simulink model "LAB_Stima_e_Controllo_Lez_5_Pendolo_Inverso_Simulink"  (R2018a)
settings: Solver=VariableStepAuto  StartTime=0.0  StopTime=10.0  RelTol=1e-3
values from neighbouring files (symbols this model uses):
  g = 9.81    [LAB_Stima_e_Controllo_Lez_2_Sistema_Idraulico.m]    (also in LAB_Stima_e_Controllo_Lez_4_Pendolo_Inverso.m)
  K2 = place(A,B,p2)    [LAB_Stima_e_Controllo_Lez_1_Motore_Corrente_Continua.m]    (also in LAB_Stima_e_Controllo_Lez_2_Sistema_Idraulico.m)
  L = KD'    [LAB_Stima_e_Controllo_Lez_2_Sistema_Idraulico.m]    (also in LAB_Stima_e_Controllo_Lez_4_Pendolo_Inverso.m = 0.5)
  m = 0.2    [LAB_Stima_e_Controllo_Lez_4_Pendolo_Inverso.m]
  M = 0.3    [LAB_Stima_e_Controllo_Lez_4_Pendolo_Inverso.m]
settings Model: Creator=anton  LastModifiedBy=anton

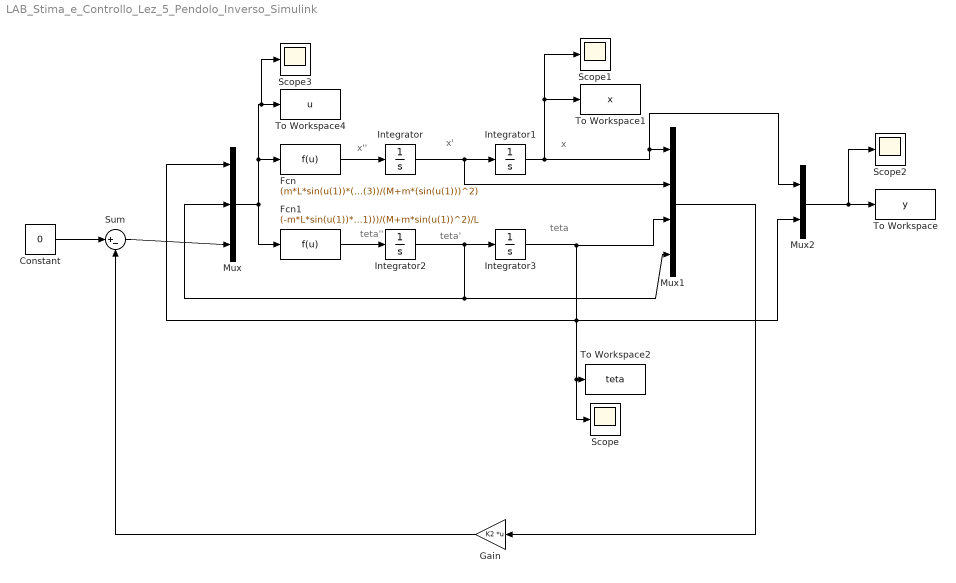
== system LAB_Stima_e_Controllo_Lez_5_Pendolo_Inverso_Simulink ==
  note: teta
  note: x
  note: teta'
  note: teta''
  note: x'
  note: x''
  Constant : Constant  Value=0
  Fcn : Fcn  Expr=(m*L*sin(u(1))*(u(2))^2-m*g*sin(u(1))*cos(u(1))+u(3))/(M+m*(sin(u(1)))^2)
  Fcn1 : Fcn  Expr=(-m*L*sin(u(1))*cos(u(1))*(u(2))^2+(M+m)*g*sin(u(1))-u(3)*cos(u(1)))/(M+m*sin(u(1))^2)/L
  Gain : Gain  Gain=K2  Multiplication=Matrix(K*u)
  Integrator : Integrator
  Integrator1 : Integrator
  Integrator2 : Integrator
  Integrator3 : Integrator  InitialCondition=0.45
  Mux : Mux  Inputs=3
  Mux1 : Mux
  Mux2 : Mux  Inputs=2
  Scope{,1..3} (4 alike) : Scope
  Sum : Sum  Inputs=|+-
  To Workspace : ToWorkspace  VariableName=y  SampleTime=-1
  To Workspace1 : ToWorkspace  VariableName=x  SampleTime=-1
  To Workspace2 : ToWorkspace  VariableName=teta  SampleTime=-1
  To Workspace4 : ToWorkspace  VariableName=u  SampleTime=-1
  wires:
  Fcn/1 -> Integrator/1
  Integrator/1 -> Mux1/2, Integrator1/1
  Fcn1/1 -> Integrator2/1
  Integrator2/1 -> Mux1/4, Mux/2, Integrator3/1
  Mux/1 -> Fcn1/1, Scope3/1, To Workspace4/1, Fcn/1
  Integrator3/1 -> Mux2/2, Scope/1, To Workspace2/1, Mux/1, Mux1/3
  Constant/1 -> Sum/1
  Sum/1 -> Mux/3
  Integrator1/1 -> Scope1/1, To Workspace1/1, Mux2/1, Mux1/1
  Mux1/1 -> Gain/1
  Gain/1 -> Sum/2
  Mux2/1 -> Scope2/1, To Workspace/1
